simulink model "CONTROL_HOLIST_ID"  (R2025b)
settings: Solver=VariableStepAuto  StartTime=0.0  StopTime=10.0  RelTol=1e-3
libraries: SCR x3
settings Model: Creator=Michael  LastModifiedBy=Michael

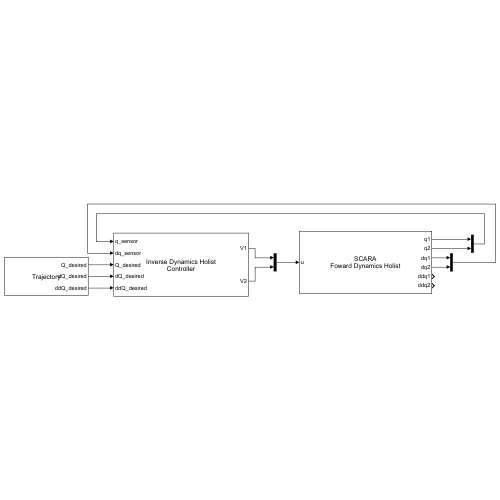
[thumbnail: Simulink's stored preview of the top-level diagram]
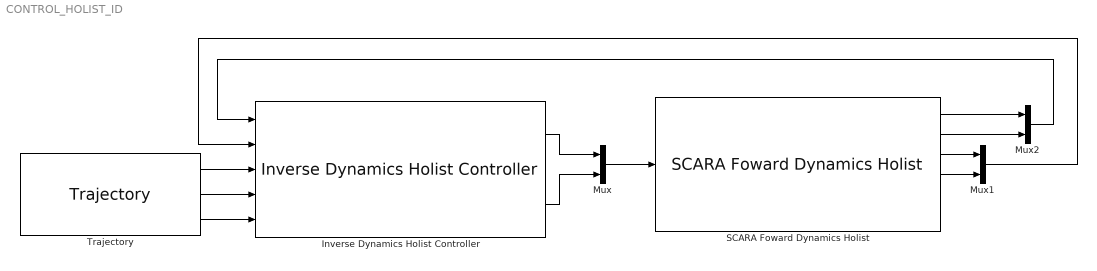
== system CONTROL_HOLIST_ID ==
  Inverse Dynamics Holist Controller : SCR/Inverse Dynamics Holist Controller  SystemSampleTime=-1  VariantActivationTime=update diagram  EmptyChoice=off  PassThrough=off  PassThroughVariantControl=(default)  EmptyChoiceVariantControl=(default)  AllowFlexibleInterface=on  Latency=0  AutoFrameSizeCalculation=off
  Mux : Mux  Inputs=2
  Mux1 : Mux  Inputs=2
  Mux2 : Mux  Inputs=2
  SCARA Foward Dynamics Holist : SCR/SCARA Foward Dynamics Holist  SystemSampleTime=-1  VariantActivationTime=update diagram  EmptyChoice=off  PassThrough=off  PassThroughVariantControl=(default)  EmptyChoiceVariantControl=(default)  AllowFlexibleInterface=on  Latency=0  AutoFrameSizeCalculation=off
  Trajectory : SCR/Trajectory  SystemSampleTime=-1  VariantActivationTime=update diagram  EmptyChoice=off  PassThrough=off  PassThroughVariantControl=(default)  EmptyChoiceVariantControl=(default)  AllowFlexibleInterface=on  Latency=0  AutoFrameSizeCalculation=off
  wires:
  Trajectory/1 -> Inverse Dynamics Holist Controller/3
  Inverse Dynamics Holist Controller/1 -> Mux/1
  Inverse Dynamics Holist Controller/2 -> Mux/2
  Mux/1 -> SCARA Foward Dynamics Holist/1
  SCARA Foward Dynamics Holist/1 -> Mux2/1
  SCARA Foward Dynamics Holist/2 -> Mux2/2
  SCARA Foward Dynamics Holist/3 -> Mux1/1
  SCARA Foward Dynamics Holist/4 -> Mux1/2
  Mux2/1 -> Inverse Dynamics Holist Controller/1
  Mux1/1 -> Inverse Dynamics Holist Controller/2
  Trajectory/3 -> Inverse Dynamics Holist Controller/5
  Trajectory/2 -> Inverse Dynamics Holist Controller/4
